simulink model "bin1_sandbox_model"  (R2020b)
settings: Solver=FixedStepDiscrete  StartTime=0.0  StopTime=2  FixedStep=0.1  RelTol=1e-3
libraries: simulink x4
settings Model: Creator=cbeal  LastModifiedBy=cbeal
settings DataIOCC: ReturnWorkspaceOutputs=off

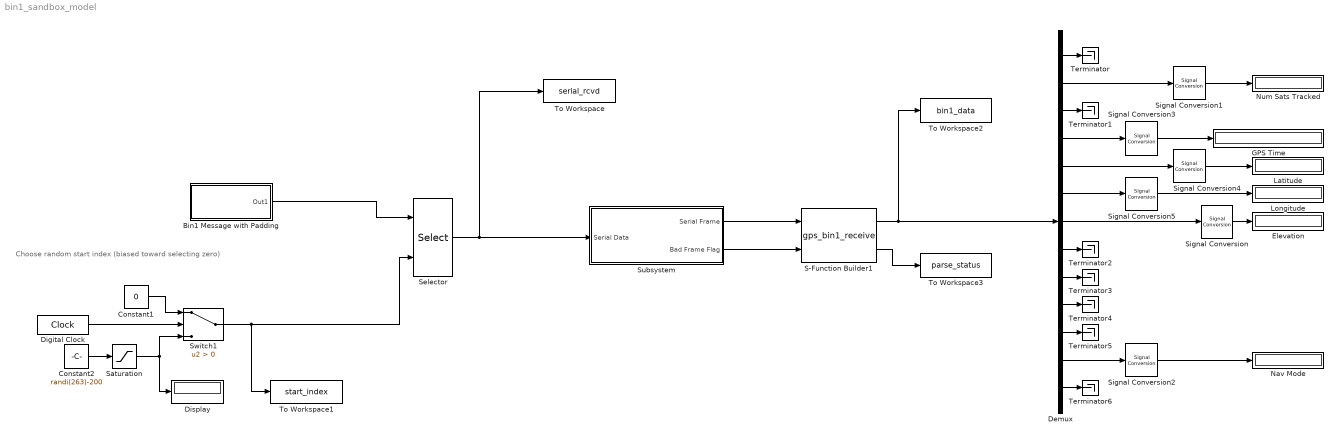
== system bin1_sandbox_model ==
  note: Choose random start index
      | (biased toward selecting zero)
  Bin1 Message with Padding : Subsystem
  Constant1 : Constant  Value=0
  Constant2 : Constant  Value=randi(263)-200
  Demux : Demux  Outputs=13
  Digital Clock : DigitalClock  SampleTime=-1
  Display : Display
  Elevation : Display
  GPS Time : Display
      settings: Format=long_e
  Latitude : Display
  Longitude : Display
  Nav Mode : Display
  Num Sats Tracked : Display
  S-Function Builder1 : S-Function  FunctionName=gps_bin1_receive  SFunctionModules=gps_bin1_receive_wrapper  SFunctionDeploymentMode=off  EnableBusSupport=off  mask(S-Function Builder){}
      mask help: Simulink:masks:SFunctionBuilder_MD
      mask init:
      | val = [[.9  0.75 0.75 1 1 .9 .9 1]',[1 1 0.75 0.75 .9 .9 1 .9]'];try , sys = get_param(gcb,'SfunBuilderFcnName');if isempty(sys), sys = get_param(gcb,'FunctionName'); end,catch, sys = get_param(gcb,'FunctionName'); end
      settings: CopyFcn=set_param(gcbh,'LinkStatus','none')  OpenFcn=sfunctionwizard(gcbh)
      mask Display:
      | plot(val(:,1),val(:,2))
      | disp(sys)
      | port_label('input',1,'u0')
      | port_label('input',2,'u1')
      | port_label('output',1,'y0')
      | port_label('output',2,'y1')
  Saturation : Saturate  UpperLimit=inf  LowerLimit=0
  Selector : Selector  IndexMode=Zero-based  InputPortWidth=164  IndexOptions=Starting index (port)  Indices=[1 3]  OutputSizes=100
  Signal Conversion{,1..5} (6 alike) : SignalConversion  OverrideOpt=off
  Subsystem : Subsystem
  Switch1 : Switch  Criteria=u2 > Threshold
  Terminator{,1..6} (7 alike) : Terminator
  To Workspace : ToWorkspace  VariableName=serial_rcvd  SampleTime=-1
      settings: Save2DSignal=2-D array (concatenate along first dimension)
  To Workspace1 : ToWorkspace  VariableName=start_index  SampleTime=-1
      settings: Save2DSignal=2-D array (concatenate along first dimension)
  To Workspace2 : ToWorkspace  VariableName=bin1_data  SampleTime=-1
      settings: Save2DSignal=2-D array (concatenate along first dimension)
  To Workspace3 : ToWorkspace  VariableName=parse_status  SampleTime=-1
      settings: Save2DSignal=2-D array (concatenate along first dimension)
  wires:
  Bin1 Message with Padding/1(Out1) -> Selector/1
  Selector/1 -> Subsystem/1(Serial Data), To Workspace/1
  S-Function Builder1/2 -> To Workspace3/1
  Switch1/1 -> Selector/2, To Workspace1/1
  Subsystem/1(Serial Frame) -> S-Function Builder1/1
  Digital Clock/1 -> Switch1/2
  Constant1/1 -> Switch1/1
  Constant2/1 -> Saturation/1
  Subsystem/2(Bad Frame Flag) -> S-Function Builder1/2
  Saturation/1 -> Display/1, Switch1/3
  S-Function Builder1/1 -> Demux/1, To Workspace2/1
  Signal Conversion5/1 -> Longitude/1
  Demux/3 -> Terminator1/1
  Demux/12 -> Signal Conversion2/1
  Demux/4 -> Signal Conversion3/1
  Demux/6 -> Signal Conversion5/1
  Demux/2 -> Signal Conversion1/1
  Demux/5 -> Signal Conversion4/1
  Demux/8 -> Terminator2/1
  Demux/7 -> Signal Conversion/1
  Demux/11 -> Terminator5/1
  Demux/1 -> Terminator/1
  Demux/9 -> Terminator3/1
  Signal Conversion3/1 -> GPS Time/1
  Signal Conversion/1 -> Elevation/1
  Signal Conversion1/1 -> Num Sats Tracked/1
  Signal Conversion4/1 -> Latitude/1
  Demux/13 -> Terminator6/1
  Demux/10 -> Terminator4/1
  Signal Conversion2/1 -> Nav Mode/1

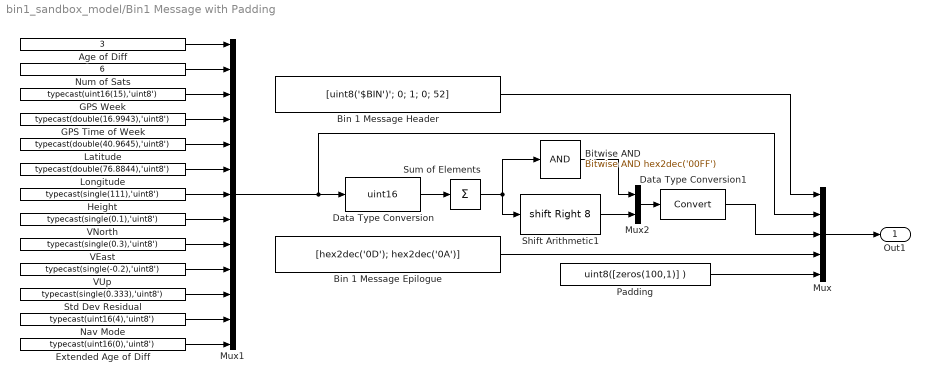
== system bin1_sandbox_model/Bin1 Message with Padding ==
  Age of Diff : Constant  Value=3  OutDataTypeStr=uint8
  Bin 1 Message Epilogue : Constant  Value=[hex2dec('0D'); hex2dec('0A')]  OutDataTypeStr=uint8
  Bin 1 Message Header : Constant  Value=[uint8('$BIN')'; 0; 1; 0; 52]
  Bitwise AND : simulink/Logic and Bit Operations/Bitwise Operator  logicop=AND  UseBitMask=on  BitMask=hex2dec('00FF')  BitMaskRealWorld=Stored Integer
  Data Type Conversion : DataTypeConversion  OutDataTypeStr=uint16
  Data Type Conversion1 : DataTypeConversion  ConvertRealWorld=Stored Integer (SI)
  Extended Age of Diff : Constant  Value=typecast(uint16(0),'uint8')  OutDataTypeStr=uint8
  GPS Time of Week : Constant  Value=typecast(double(16.9943),'uint8')  OutDataTypeStr=uint8
  GPS Week : Constant  Value=typecast(uint16(15),'uint8')  OutDataTypeStr=uint8
  Height : Constant  Value=typecast(single(111),'uint8')  OutDataTypeStr=uint8
  Latitude : Constant  Value=typecast(double(40.9645),'uint8')  OutDataTypeStr=uint8
  Longitude : Constant  Value=typecast(double(76.8844),'uint8')  OutDataTypeStr=uint8
  Mux : Mux  Inputs=5
  Mux1 : Mux  Inputs=13
  Mux2 : Mux  Inputs=2
  Nav Mode : Constant  Value=typecast(uint16(4),'uint8')  OutDataTypeStr=uint8
  Num of Sats : Constant  Value=6  OutDataTypeStr=uint8
  Padding : Constant  Value=uint8([zeros(100,1)] )
  Shift Arithmetic1 : ArithShift  BitShiftNumber=8  BitShiftDirection=Right
  Std Dev Residual : Constant  Value=typecast(single(0.333),'uint8')  OutDataTypeStr=uint8
  Sum of Elements : Sum  Inputs=+  AccumDataTypeStr=uint16  OutDataTypeStr=uint16
  VEast : Constant  Value=typecast(single(0.3),'uint8')  OutDataTypeStr=uint8
  VNorth : Constant  Value=typecast(single(0.1),'uint8')  OutDataTypeStr=uint8
  VUp : Constant  Value=typecast(single(-0.2),'uint8')  OutDataTypeStr=uint8
  Out1 : Outport
  wires:
  Padding/1 -> Mux/5
  Bin 1 Message Header/1 -> Mux/1
  Mux/1 -> Out1/1
  Bin 1 Message Epilogue/1 -> Mux/4
  Data Type Conversion/1 -> Sum of Elements/1
  Mux1/1 -> Mux/2, Data Type Conversion/1
  Age of Diff/1 -> Mux1/1
  Num of Sats/1 -> Mux1/2
  GPS Week/1 -> Mux1/3
  GPS Time of Week/1 -> Mux1/4
  Latitude/1 -> Mux1/5
  Longitude/1 -> Mux1/6
  Height/1 -> Mux1/7
  VNorth/1 -> Mux1/8
  VEast/1 -> Mux1/9
  VUp/1 -> Mux1/10
  Std Dev Residual/1 -> Mux1/11
  Nav Mode/1 -> Mux1/12
  Extended Age of Diff/1 -> Mux1/13
  Data Type Conversion1/1 -> Mux/3
  Sum of Elements/1 -> Bitwise AND/1, Shift Arithmetic1/1
  Shift Arithmetic1/1 -> Mux2/2
  Mux2/1 -> Data Type Conversion1/1
  Bitwise AND/1 -> Mux2/1

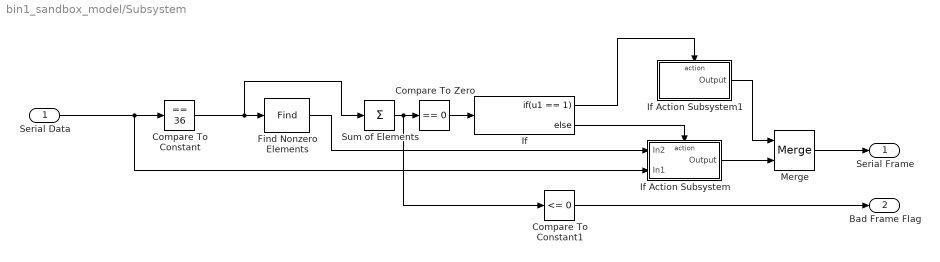
== system bin1_sandbox_model/Subsystem ==
  Serial Data : Inport
  Compare To Constant : simulink/Logic and Bit Operations/Compare To Constant  relop===  const=36  OutDataTypeStr=boolean
  Compare To Constant1 : simulink/Logic and Bit Operations/Compare To Constant  relop=<=  const=0  OutDataTypeStr=uint8
  Compare To Zero : simulink/Logic and Bit Operations/Compare To Zero  relop===  OutDataTypeStr=boolean
  Find Nonzero Elements : Find  NumberOfInputDimensions=3
  If : If  IfExpression=u1 == 1
  If Action Subsystem : Subsystem  TreatAsAtomicUnit=on
  If Action Subsystem1 : Subsystem  TreatAsAtomicUnit=on
  Merge : Merge
  Sum of Elements : Sum  Inputs=+
  Serial Frame : Outport
  Bad Frame Flag : Outport  Port=2
  wires:
  Compare To Constant1/1 -> Bad Frame Flag/1
  Find Nonzero Elements/1 -> If Action Subsystem/1(In2)
  Sum of Elements/1 -> Compare To Constant1/1, Compare To Zero/1
  If Action Subsystem1/1(Output) -> Merge/1
  Compare To Constant/1 -> Sum of Elements/1, Find Nonzero Elements/1
  Compare To Zero/1 -> If/1
  If/1 -> If Action Subsystem1/Action
  If/2 -> If Action Subsystem/Action
  If Action Subsystem/1(Output) -> Merge/2
  Serial Data/1 -> If Action Subsystem/2(In1), Compare To Constant/1
  Merge/1 -> Serial Frame/1

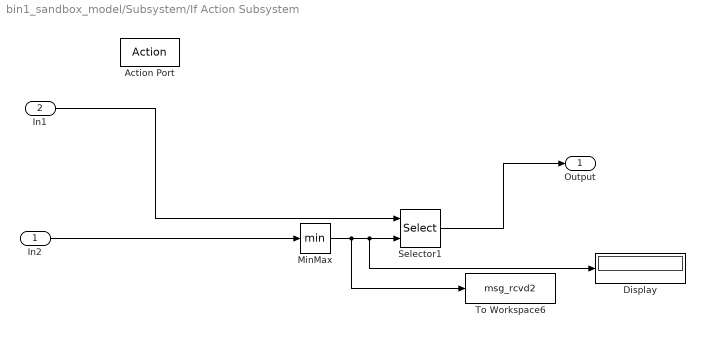
== system bin1_sandbox_model/Subsystem/If Action Subsystem ==
  In2 : Inport
  In1 : Inport  Port=2
  Action Port : ActionPort  ActionPortLabel=else
  Display : Display
  MinMax : MinMax
  Selector1 : Selector  InputPortWidth=100  IndexOptions=Starting index (port)  Indices=[1 3]  OutputSizes=64
  To Workspace6 : ToWorkspace  VariableName=msg_rcvd2  SampleTime=-1
      settings: Save2DSignal=2-D array (concatenate along first dimension)
  Output : Outport
  wires:
  Selector1/1 -> Output/1
  In1/1 -> Selector1/1
  MinMax/1 -> Selector1/2, Display/1, To Workspace6/1
  In2/1 -> MinMax/1

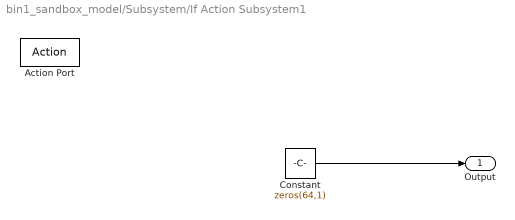
== system bin1_sandbox_model/Subsystem/If Action Subsystem1 ==
  Action Port : ActionPort  ActionPortLabel=if(u1 == 1)
  Constant : Constant  Value=zeros(64,1)  OutDataTypeStr=uint8
  Output : Outport
  wires:
  Constant/1 -> Output/1
